simulink model "ProiectSCPC_Reglare_Nivel"  (R2023a)
settings: Solver=FixedStepAuto  StartTime=0.0  StopTime=1000  FixedStep=0.01  RelTol=1e-3
undefined symbols (not defined in the file): C, k, k1, k11, k12, k13, k2, k3, keta
libraries: slpidlib x8
settings Model: Creator=Cristian  LastModifiedBy=Cristian

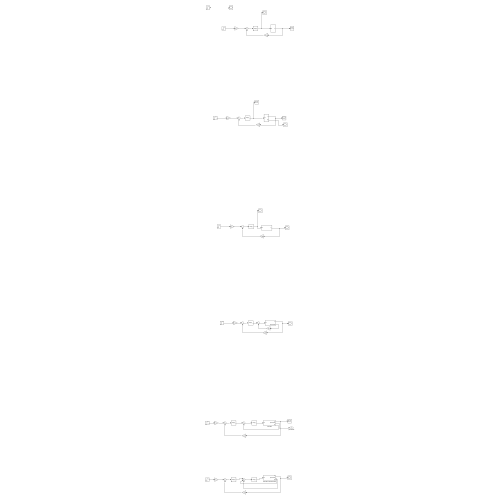
[thumbnail: Simulink's stored preview of the top-level diagram]
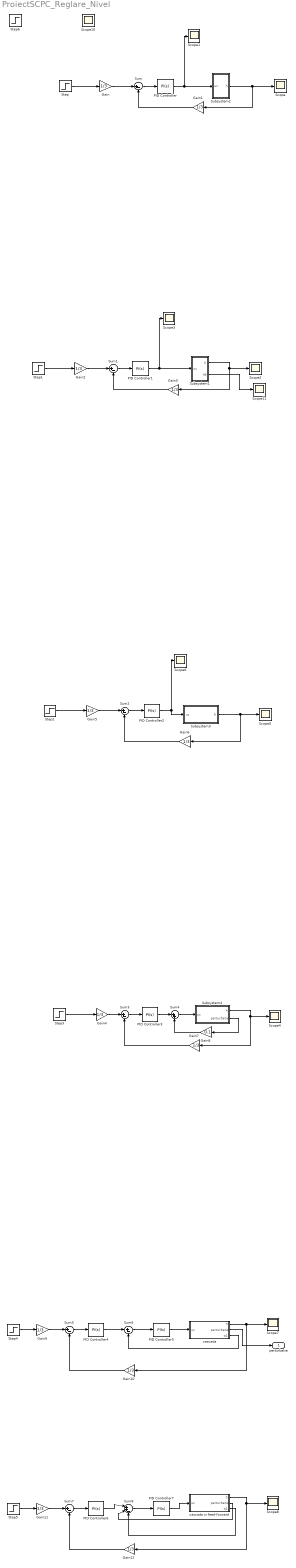
== system ProiectSCPC_Reglare_Nivel ==
  Gain{,1..7,9..12} (12 alike) : Gain  Gain=1/3
  Gain8 : Gain  Gain=0.1
  PID Controller{,1..3} (4 alike) : slpidlib/PID Controller  Controller=PI  Form=Parallel  TimeDomain=Continuous-time  UseExternalTs=off  SampleTime=-1  IntegratorMethod=Forward Euler  FilterMethod=Forward Euler  ControllerParametersSource=internal  P=2.395  I=2.395/160  UseKiTs=off  D=0  N=100  UseFilter=on  TunerSelectOption=Transfer Function Based (PID Tuner App)  InitialConditionSource=internal  InitialConditionForIntegrator=5  InitialConditionForFilter=0  DifferentiatorICPrevScaledInput=0  ExternalReset=none  TrackingMode=off  Kt=1  LimitOutput=off  SatLimitsSource=internal  UpperSaturationLimit=inf  LowerSaturationLimit=-inf  LinearizeAsGain=on  AntiWindupMode=none  Kb=1  LimitIntegrator=off  UpperIntegratorSaturationLimit=inf  LowerIntegratorSaturationLimit=-inf  POutMin=[]  POutMax=[]  IOutMin=[]  IOutMax=[]  DOutMin=[]  DOutMax=[]  NOutMin=[]  NOutMax=[]  SumOutMin=[]  SumOutMax=[]  SaturationOutMin=[]  SaturationOutMax=[]  PParamMin=[]  PParamMax=[]  IParamMin=[]  IParamMax=[]  DParamMin=[]  DParamMax=[]  NParamMin=[]  NParamMax=[]  KbParamMin=[]  KbParamMax=[]  KtParamMin=[]  KtParamMax=[]  KbOutMin=[]  KbOutMax=[]  KtOutMin=[]  KtOutMax=[]  IntegratorOutMin=[]  IntegratorOutMax=[]  FilterOutMin=[]  FilterOutMax=[]  SumI1OutMin=[]  SumI1OutMax=[]  SumI2OutMin=[]  SumI2OutMax=[]  SumI3OutMin=[]  SumI3OutMax=[]  SumI4OutMin=[]  SumI4OutMax=[]  SumDOutMin=[]  SumDOutMax=[]  DifferentiatorOutMin=[]  DifferentiatorOutMax=[]  FilterDiffOutCoefMin=[]  FilterDiffOutCoefMax=[]  ReciprocalOutMin=[]  ReciprocalOutMax=[]  SumDenOutMin=[]  SumDenOutMax=[]  SumNumOutMin=[]  SumNumOutMax=[]  DivideOutMin=[]  DivideOutMax=[]  UdiffTsProdOutMin=[]  UdiffTsProdOutMax=[]  NTsProdOutMin=[]  NTsProdOutMax=[]  UintegralTsProdOutMin=[]  UintegralTsProdOutMax=[]  UngainTsProdOutMin=[]  UngainTsProdOutMax=[]  ClampingZeroOutDataTypeStr=Inherit: Inherit via back propagation  ClampingZeroOutMin=[]  ClampingZeroOutMax=[]  FilterDenConstantOutDataTypeStr=Inherit: Inherit via back propagation  FilterDenConstantOutMin=[]  FilterDenConstantOutMax=[]  PCopyOutDataTypeStr=Inherit: Inherit via back propagation  PCopyOutMin=[]  PCopyOutMax=[]  NCopyOutDataTypeStr=Inherit: Inherit via back propagation  NCopyOutMin=[]  NCopyOutMax=[]  IntegratorContinuousStateAttributes=''  IntegratorStateMustResolveToSignalObject=off  IntegratorRTWStateStorageClass=Auto  FilterContinuousStateAttributes=''  FilterStateMustResolveToSignalObject=off  FilterRTWStateStorageClass=Auto  ParallelPVariant=InternalParameters  IdealPVariant=Disabled  IVariant=InternalParameters  DVariant=Disabled  IntegratorVariant=Continuous  SatVariant=Disabled  AWVariant=Passthrough  PCopyVariant=Disabled  TRVariant=Disabled  FdbkBlocksVariant=Forward  IdealPFdbkVariant=Disabled  SatFdbkVariant=Disabled  DerivativeFilterVariant=Disabled  NVariant=Disabled  NCopyVariant=Disabled_SignalSpec  FilterICVariant=Disabled  IntegratorICVariant=InternalICs  ExternalResetVariant=Disabled  TRSumVariant=Passthrough  SumFdbkVariant=Disabled  SumVariant=Sum_PI  TsampFilterVariant=InternalTs  TsampNgainVariant=Passthrough  TsampIntegralVariant=Disabled_SignalSpec  ExternalSaturationOutDataTypeStr=Inherit: Same as second input
  PID Controller4 : slpidlib/PID Controller  Controller=PI  Form=Parallel  TimeDomain=Continuous-time  UseExternalTs=off  SampleTime=-1  IntegratorMethod=Forward Euler  FilterMethod=Forward Euler  ControllerParametersSource=internal  P=39  I=0.16  UseKiTs=off  D=0  N=100  UseFilter=on  TunerSelectOption=Transfer Function Based (PID Tuner App)  InitialConditionSource=internal  InitialConditionForIntegrator=29.2  InitialConditionForFilter=0  DifferentiatorICPrevScaledInput=0  ExternalReset=none  TrackingMode=off  Kt=1  LimitOutput=off  SatLimitsSource=internal  UpperSaturationLimit=inf  LowerSaturationLimit=-inf  LinearizeAsGain=on  AntiWindupMode=none  Kb=1  LimitIntegrator=off  UpperIntegratorSaturationLimit=inf  LowerIntegratorSaturationLimit=-inf  POutMin=[]  POutMax=[]  IOutMin=[]  IOutMax=[]  DOutMin=[]  DOutMax=[]  NOutMin=[]  NOutMax=[]  SumOutMin=[]  SumOutMax=[]  SaturationOutMin=[]  SaturationOutMax=[]  PParamMin=[]  PParamMax=[]  IParamMin=[]  IParamMax=[]  DParamMin=[]  DParamMax=[]  NParamMin=[]  NParamMax=[]  KbParamMin=[]  KbParamMax=[]  KtParamMin=[]  KtParamMax=[]  KbOutMin=[]  KbOutMax=[]  KtOutMin=[]  KtOutMax=[]  IntegratorOutMin=[]  IntegratorOutMax=[]  FilterOutMin=[]  FilterOutMax=[]  SumI1OutMin=[]  SumI1OutMax=[]  SumI2OutMin=[]  SumI2OutMax=[]  SumI3OutMin=[]  SumI3OutMax=[]  SumI4OutMin=[]  SumI4OutMax=[]  SumDOutMin=[]  SumDOutMax=[]  DifferentiatorOutMin=[]  DifferentiatorOutMax=[]  FilterDiffOutCoefMin=[]  FilterDiffOutCoefMax=[]  ReciprocalOutMin=[]  ReciprocalOutMax=[]  SumDenOutMin=[]  SumDenOutMax=[]  SumNumOutMin=[]  SumNumOutMax=[]  DivideOutMin=[]  DivideOutMax=[]  UdiffTsProdOutMin=[]  UdiffTsProdOutMax=[]  NTsProdOutMin=[]  NTsProdOutMax=[]  UintegralTsProdOutMin=[]  UintegralTsProdOutMax=[]  UngainTsProdOutMin=[]  UngainTsProdOutMax=[]  ClampingZeroOutDataTypeStr=Inherit: Inherit via back propagation  ClampingZeroOutMin=[]  ClampingZeroOutMax=[]  FilterDenConstantOutDataTypeStr=Inherit: Inherit via back propagation  FilterDenConstantOutMin=[]  FilterDenConstantOutMax=[]  PCopyOutDataTypeStr=Inherit: Inherit via back propagation  PCopyOutMin=[]  PCopyOutMax=[]  NCopyOutDataTypeStr=Inherit: Inherit via back propagation  NCopyOutMin=[]  NCopyOutMax=[]  IntegratorContinuousStateAttributes=''  IntegratorStateMustResolveToSignalObject=off  IntegratorRTWStateStorageClass=Auto  FilterContinuousStateAttributes=''  FilterStateMustResolveToSignalObject=off  FilterRTWStateStorageClass=Auto  ParallelPVariant=InternalParameters  IdealPVariant=Disabled  IVariant=InternalParameters  DVariant=Disabled  IntegratorVariant=Continuous  SatVariant=Disabled  AWVariant=Passthrough  PCopyVariant=Disabled  TRVariant=Disabled  FdbkBlocksVariant=Forward  IdealPFdbkVariant=Disabled  SatFdbkVariant=Disabled  DerivativeFilterVariant=Disabled  NVariant=Disabled  NCopyVariant=Disabled_SignalSpec  FilterICVariant=Disabled  IntegratorICVariant=InternalICs  ExternalResetVariant=Disabled  TRSumVariant=Passthrough  SumFdbkVariant=Disabled  SumVariant=Sum_PI  TsampFilterVariant=InternalTs  TsampNgainVariant=Passthrough  TsampIntegralVariant=Disabled_SignalSpec  ExternalSaturationOutDataTypeStr=Inherit: Same as second input
  PID Controller5 : slpidlib/PID Controller  Controller=PI  Form=Parallel  TimeDomain=Continuous-time  UseExternalTs=off  SampleTime=-1  IntegratorMethod=Forward Euler  FilterMethod=Forward Euler  ControllerParametersSource=internal  P=0.07  I=1  UseKiTs=off  D=0  N=100  UseFilter=on  TunerSelectOption=Transfer Function Based (PID Tuner App)  InitialConditionSource=internal  InitialConditionForIntegrator=5  InitialConditionForFilter=0  DifferentiatorICPrevScaledInput=0  ExternalReset=none  TrackingMode=off  Kt=1  LimitOutput=off  SatLimitsSource=internal  UpperSaturationLimit=inf  LowerSaturationLimit=-inf  LinearizeAsGain=on  AntiWindupMode=none  Kb=1  LimitIntegrator=off  UpperIntegratorSaturationLimit=inf  LowerIntegratorSaturationLimit=-inf  POutMin=[]  POutMax=[]  IOutMin=[]  IOutMax=[]  DOutMin=[]  DOutMax=[]  NOutMin=[]  NOutMax=[]  SumOutMin=[]  SumOutMax=[]  SaturationOutMin=[]  SaturationOutMax=[]  PParamMin=[]  PParamMax=[]  IParamMin=[]  IParamMax=[]  DParamMin=[]  DParamMax=[]  NParamMin=[]  NParamMax=[]  KbParamMin=[]  KbParamMax=[]  KtParamMin=[]  KtParamMax=[]  KbOutMin=[]  KbOutMax=[]  KtOutMin=[]  KtOutMax=[]  IntegratorOutMin=[]  IntegratorOutMax=[]  FilterOutMin=[]  FilterOutMax=[]  SumI1OutMin=[]  SumI1OutMax=[]  SumI2OutMin=[]  SumI2OutMax=[]  SumI3OutMin=[]  SumI3OutMax=[]  SumI4OutMin=[]  SumI4OutMax=[]  SumDOutMin=[]  SumDOutMax=[]  DifferentiatorOutMin=[]  DifferentiatorOutMax=[]  FilterDiffOutCoefMin=[]  FilterDiffOutCoefMax=[]  ReciprocalOutMin=[]  ReciprocalOutMax=[]  SumDenOutMin=[]  SumDenOutMax=[]  SumNumOutMin=[]  SumNumOutMax=[]  DivideOutMin=[]  DivideOutMax=[]  UdiffTsProdOutMin=[]  UdiffTsProdOutMax=[]  NTsProdOutMin=[]  NTsProdOutMax=[]  UintegralTsProdOutMin=[]  UintegralTsProdOutMax=[]  UngainTsProdOutMin=[]  UngainTsProdOutMax=[]  ClampingZeroOutDataTypeStr=Inherit: Inherit via back propagation  ClampingZeroOutMin=[]  ClampingZeroOutMax=[]  FilterDenConstantOutDataTypeStr=Inherit: Inherit via back propagation  FilterDenConstantOutMin=[]  FilterDenConstantOutMax=[]  PCopyOutDataTypeStr=Inherit: Inherit via back propagation  PCopyOutMin=[]  PCopyOutMax=[]  NCopyOutDataTypeStr=Inherit: Inherit via back propagation  NCopyOutMin=[]  NCopyOutMax=[]  IntegratorContinuousStateAttributes=''  IntegratorStateMustResolveToSignalObject=off  IntegratorRTWStateStorageClass=Auto  FilterContinuousStateAttributes=''  FilterStateMustResolveToSignalObject=off  FilterRTWStateStorageClass=Auto  ParallelPVariant=InternalParameters  IdealPVariant=Disabled  IVariant=InternalParameters  DVariant=Disabled  IntegratorVariant=Continuous  SatVariant=Disabled  AWVariant=Passthrough  PCopyVariant=Disabled  TRVariant=Disabled  FdbkBlocksVariant=Forward  IdealPFdbkVariant=Disabled  SatFdbkVariant=Disabled  DerivativeFilterVariant=Disabled  NVariant=Disabled  NCopyVariant=Disabled_SignalSpec  FilterICVariant=Disabled  IntegratorICVariant=InternalICs  ExternalResetVariant=Disabled  TRSumVariant=Passthrough  SumFdbkVariant=Disabled  SumVariant=Sum_PI  TsampFilterVariant=InternalTs  TsampNgainVariant=Passthrough  TsampIntegralVariant=Disabled_SignalSpec  ExternalSaturationOutDataTypeStr=Inherit: Same as second input
  PID Controller6 : slpidlib/PID Controller  Controller=PI  Form=Parallel  TimeDomain=Continuous-time  UseExternalTs=off  SampleTime=-1  IntegratorMethod=Forward Euler  FilterMethod=Forward Euler  ControllerParametersSource=internal  P=40  I=40/250  UseKiTs=off  D=0  N=100  UseFilter=on  TunerSelectOption=Transfer Function Based (PID Tuner App)  InitialConditionSource=internal  InitialConditionForIntegrator=29.2  InitialConditionForFilter=0  DifferentiatorICPrevScaledInput=0  ExternalReset=none  TrackingMode=off  Kt=1  LimitOutput=off  SatLimitsSource=internal  UpperSaturationLimit=inf  LowerSaturationLimit=-inf  LinearizeAsGain=on  AntiWindupMode=none  Kb=1  LimitIntegrator=off  UpperIntegratorSaturationLimit=inf  LowerIntegratorSaturationLimit=-inf  POutMin=[]  POutMax=[]  IOutMin=[]  IOutMax=[]  DOutMin=[]  DOutMax=[]  NOutMin=[]  NOutMax=[]  SumOutMin=[]  SumOutMax=[]  SaturationOutMin=[]  SaturationOutMax=[]  PParamMin=[]  PParamMax=[]  IParamMin=[]  IParamMax=[]  DParamMin=[]  DParamMax=[]  NParamMin=[]  NParamMax=[]  KbParamMin=[]  KbParamMax=[]  KtParamMin=[]  KtParamMax=[]  KbOutMin=[]  KbOutMax=[]  KtOutMin=[]  KtOutMax=[]  IntegratorOutMin=[]  IntegratorOutMax=[]  FilterOutMin=[]  FilterOutMax=[]  SumI1OutMin=[]  SumI1OutMax=[]  SumI2OutMin=[]  SumI2OutMax=[]  SumI3OutMin=[]  SumI3OutMax=[]  SumI4OutMin=[]  SumI4OutMax=[]  SumDOutMin=[]  SumDOutMax=[]  DifferentiatorOutMin=[]  DifferentiatorOutMax=[]  FilterDiffOutCoefMin=[]  FilterDiffOutCoefMax=[]  ReciprocalOutMin=[]  ReciprocalOutMax=[]  SumDenOutMin=[]  SumDenOutMax=[]  SumNumOutMin=[]  SumNumOutMax=[]  DivideOutMin=[]  DivideOutMax=[]  UdiffTsProdOutMin=[]  UdiffTsProdOutMax=[]  NTsProdOutMin=[]  NTsProdOutMax=[]  UintegralTsProdOutMin=[]  UintegralTsProdOutMax=[]  UngainTsProdOutMin=[]  UngainTsProdOutMax=[]  ClampingZeroOutDataTypeStr=Inherit: Inherit via back propagation  ClampingZeroOutMin=[]  ClampingZeroOutMax=[]  FilterDenConstantOutDataTypeStr=Inherit: Inherit via back propagation  FilterDenConstantOutMin=[]  FilterDenConstantOutMax=[]  PCopyOutDataTypeStr=Inherit: Inherit via back propagation  PCopyOutMin=[]  PCopyOutMax=[]  NCopyOutDataTypeStr=Inherit: Inherit via back propagation  NCopyOutMin=[]  NCopyOutMax=[]  IntegratorContinuousStateAttributes=''  IntegratorStateMustResolveToSignalObject=off  IntegratorRTWStateStorageClass=Auto  FilterContinuousStateAttributes=''  FilterStateMustResolveToSignalObject=off  FilterRTWStateStorageClass=Auto  ParallelPVariant=InternalParameters  IdealPVariant=Disabled  IVariant=InternalParameters  DVariant=Disabled  IntegratorVariant=Continuous  SatVariant=Disabled  AWVariant=Passthrough  PCopyVariant=Disabled  TRVariant=Disabled  FdbkBlocksVariant=Forward  IdealPFdbkVariant=Disabled  SatFdbkVariant=Disabled  DerivativeFilterVariant=Disabled  NVariant=Disabled  NCopyVariant=Disabled_SignalSpec  FilterICVariant=Disabled  IntegratorICVariant=InternalICs  ExternalResetVariant=Disabled  TRSumVariant=Passthrough  SumFdbkVariant=Disabled  SumVariant=Sum_PI  TsampFilterVariant=InternalTs  TsampNgainVariant=Passthrough  TsampIntegralVariant=Disabled_SignalSpec  ExternalSaturationOutDataTypeStr=Inherit: Same as second input
  PID Controller7 : slpidlib/PID Controller  Controller=PI  Form=Parallel  TimeDomain=Continuous-time  UseExternalTs=off  SampleTime=-1  IntegratorMethod=Forward Euler  FilterMethod=Forward Euler  ControllerParametersSource=internal  P=0.07  I=1  UseKiTs=off  D=0  N=100  UseFilter=on  TunerSelectOption=Transfer Function Based (PID Tuner App)  InitialConditionSource=internal  InitialConditionForIntegrator=5  InitialConditionForFilter=0  DifferentiatorICPrevScaledInput=0  ExternalReset=none  TrackingMode=off  Kt=1  LimitOutput=off  SatLimitsSource=internal  UpperSaturationLimit=inf  LowerSaturationLimit=-inf  LinearizeAsGain=on  AntiWindupMode=none  Kb=1  LimitIntegrator=off  UpperIntegratorSaturationLimit=inf  LowerIntegratorSaturationLimit=-inf  POutMin=[]  POutMax=[]  IOutMin=[]  IOutMax=[]  DOutMin=[]  DOutMax=[]  NOutMin=[]  NOutMax=[]  SumOutMin=[]  SumOutMax=[]  SaturationOutMin=[]  SaturationOutMax=[]  PParamMin=[]  PParamMax=[]  IParamMin=[]  IParamMax=[]  DParamMin=[]  DParamMax=[]  NParamMin=[]  NParamMax=[]  KbParamMin=[]  KbParamMax=[]  KtParamMin=[]  KtParamMax=[]  KbOutMin=[]  KbOutMax=[]  KtOutMin=[]  KtOutMax=[]  IntegratorOutMin=[]  IntegratorOutMax=[]  FilterOutMin=[]  FilterOutMax=[]  SumI1OutMin=[]  SumI1OutMax=[]  SumI2OutMin=[]  SumI2OutMax=[]  SumI3OutMin=[]  SumI3OutMax=[]  SumI4OutMin=[]  SumI4OutMax=[]  SumDOutMin=[]  SumDOutMax=[]  DifferentiatorOutMin=[]  DifferentiatorOutMax=[]  FilterDiffOutCoefMin=[]  FilterDiffOutCoefMax=[]  ReciprocalOutMin=[]  ReciprocalOutMax=[]  SumDenOutMin=[]  SumDenOutMax=[]  SumNumOutMin=[]  SumNumOutMax=[]  DivideOutMin=[]  DivideOutMax=[]  UdiffTsProdOutMin=[]  UdiffTsProdOutMax=[]  NTsProdOutMin=[]  NTsProdOutMax=[]  UintegralTsProdOutMin=[]  UintegralTsProdOutMax=[]  UngainTsProdOutMin=[]  UngainTsProdOutMax=[]  ClampingZeroOutDataTypeStr=Inherit: Inherit via back propagation  ClampingZeroOutMin=[]  ClampingZeroOutMax=[]  FilterDenConstantOutDataTypeStr=Inherit: Inherit via back propagation  FilterDenConstantOutMin=[]  FilterDenConstantOutMax=[]  PCopyOutDataTypeStr=Inherit: Inherit via back propagation  PCopyOutMin=[]  PCopyOutMax=[]  NCopyOutDataTypeStr=Inherit: Inherit via back propagation  NCopyOutMin=[]  NCopyOutMax=[]  IntegratorContinuousStateAttributes=''  IntegratorStateMustResolveToSignalObject=off  IntegratorRTWStateStorageClass=Auto  FilterContinuousStateAttributes=''  FilterStateMustResolveToSignalObject=off  FilterRTWStateStorageClass=Auto  ParallelPVariant=InternalParameters  IdealPVariant=Disabled  IVariant=InternalParameters  DVariant=Disabled  IntegratorVariant=Continuous  SatVariant=Disabled  AWVariant=Passthrough  PCopyVariant=Disabled  TRVariant=Disabled  FdbkBlocksVariant=Forward  IdealPFdbkVariant=Disabled  SatFdbkVariant=Disabled  DerivativeFilterVariant=Disabled  NVariant=Disabled  NCopyVariant=Disabled_SignalSpec  FilterICVariant=Disabled  IntegratorICVariant=InternalICs  ExternalResetVariant=Disabled  TRSumVariant=Passthrough  SumFdbkVariant=Disabled  SumVariant=Sum_PI  TsampFilterVariant=InternalTs  TsampNgainVariant=Passthrough  TsampIntegralVariant=Disabled_SignalSpec  ExternalSaturationOutDataTypeStr=Inherit: Same as second input
  Scope{,1..8,10..11} (11 alike) : Scope
  Step{,1..3} (4 alike) : Step  Time=0  Before=10.5  After=13  SampleTime=0
  Step4 : Step  Before=10.51  After=13  SampleTime=0
  Step5 : Step  Before=10.51  After=13  SampleTime=0
  Step6 : Step  Time=0  Before=5  After=5.5  SampleTime=0
  Subsystem1 : Subsystem
  Subsystem2 : Subsystem
  Subsystem3 : Subsystem
  Subsystem4 : Subsystem
  Sum{,1..3,5..7} (7 alike) : Sum  Inputs=|+-
  Sum4 : Sum  Inputs=|++
  Sum8 : Sum  Inputs=|++-
  cascada : Subsystem
  cascada si feed-forward : Subsystem
  perturbatie : Outport
  wires:
  Subsystem2/1(h) -> Gain1/1, Scope/1
  Gain/1 -> Sum/1
  Sum/1 -> PID Controller/1
  Gain1/1 -> Sum/2
  PID Controller/1 -> Subsystem2/1(uc), Scope1/1
  Step/1 -> Gain/1
  Sum1/1 -> PID Controller1/1
  Step1/1 -> Gain2/1
  Subsystem1/2(qe) -> Scope11/1
  Subsystem1/1(h) -> Gain3/1, Scope2/1
  Gain3/1 -> Sum1/2
  PID Controller1/1 -> Subsystem1/1(uc), Scope3/1
  Gain2/1 -> Sum1/1
  PID Controller2/1 -> Scope6/1, Subsystem3/1(uc)
  Gain6/1 -> Sum2/2
  Sum2/1 -> PID Controller2/1
  Sum3/1 -> PID Controller3/1
  Subsystem4/1(h) -> Gain7/1, Scope4/1
  Step2/1 -> Gain5/1
  Gain7/1 -> Sum3/2
  Step3/1 -> Gain4/1
  PID Controller3/1 -> Sum4/1
  Subsystem4/2(perturbatie) -> Gain8/1
  Gain5/1 -> Sum2/1
  Gain8/1 -> Sum4/2
  Sum4/1 -> Subsystem4/1(uc)
  Subsystem3/1(h) -> Scope5/1, Gain6/1
  Gain4/1 -> Sum3/1
  cascada/1("h ") -> Scope7/1, Gain10/1
  PID Controller4/1 -> Sum6/1
  PID Controller5/1 -> cascada/1(uc)
  Gain10/1 -> Sum5/2
  Gain9/1 -> Sum5/1
  Step4/1 -> Gain9/1
  cascada/3(q1) -> Sum6/2
  Sum6/1 -> PID Controller5/1
  Sum5/1 -> PID Controller4/1
  cascada/2(perturbatie) -> perturbatie/1
  Gain12/1 -> Sum7/2
  cascada si feed-forward/2(perturbatie) -> Sum8/2
  Gain11/1 -> Sum7/1
  Sum7/1 -> PID Controller6/1
  Sum8/1 -> PID Controller7/1
  Step5/1 -> Gain11/1
  cascada si feed-forward/3(q1) -> Sum8/3
  cascada si feed-forward/1("h ") -> Scope8/1, Gain12/1
  PID Controller7/1 -> cascada si feed-forward/1(uc)
  PID Controller6/1 -> Sum8/1

== system ProiectSCPC_Reglare_Nivel/Subsystem1 ==
  uc : Inport
  Amplificator : Subsystem
  Bazin : Subsystem
  Curent : Subsystem
  Motor : Subsystem
  Pompa : Subsystem
  Randament : Subsystem
  Subsystem : Subsystem
  h : Outport
  qe : Outport  Port=2
  wires:
  Randament/1(eta) -> Curent/3(eta)
  Subsystem/1(h) -> Bazin/1(q), Randament/1(q), Curent/2(q)
  Amplificator/1(um) -> Curent/4(um), Randament/2(um), Motor/1(um)
  uc/1 -> Amplificator/1(ua)
  Curent/1(im) -> Motor/2(im)
  Bazin/1(h) -> h/1, Curent/1(h), Pompa/2(h)
  Motor/1(kn) -> Pompa/1(kn)
  Pompa/1(q) -> Subsystem/1(q)
  Bazin/2(qe) -> qe/1

== system ProiectSCPC_Reglare_Nivel/Subsystem2 ==
  uc : Inport
  Amplificator : Subsystem
  Bazin : Subsystem
  Curent : Subsystem
  Motor : Subsystem
  Pompa : Subsystem
  Randament : Subsystem
  Subsystem : Subsystem
  h : Outport
  wires:
  Randament/1(eta) -> Curent/3(eta)
  Subsystem/1(h) -> Bazin/1(q), Randament/1(q), Curent/2(q)
  Amplificator/1(um) -> Curent/4(um), Randament/2(um), Motor/1(um)
  uc/1 -> Amplificator/1(ua)
  Curent/1(im) -> Motor/2(im)
  Bazin/1(h) -> h/1, Curent/1(h), Pompa/2(h)
  Motor/1(kn) -> Pompa/1(kn)
  Pompa/1(q) -> Subsystem/1(q)

== system ProiectSCPC_Reglare_Nivel/Subsystem3 ==
  uc : Inport
  Amplificator : Subsystem
  Bazin : Subsystem
  Curent : Subsystem
  Motor : Subsystem
  Pompa : Subsystem
  Randament : Subsystem
  Step : Step  Time=250  After=0.01  SampleTime=0
  Subsystem : Subsystem
  h : Outport
  wires:
  Motor/1(kn) -> Pompa/1(kn1)
  Subsystem/1(h) -> Bazin/1(q), Randament/1(q), Curent/2(q)
  Pompa/1(q1) -> Subsystem/1(q)
  Randament/1(eta) -> Curent/3(eta)
  Curent/1(im) -> Motor/2(im)
  Bazin/1(h) -> h/1, Pompa/3(h1), Curent/1(h)
  uc/1 -> Amplificator/1(ua)
  Amplificator/1(um) -> Curent/4(um), Randament/2(um), Motor/1(um)
  Step/1 -> Pompa/2(perturbatie k)

== system ProiectSCPC_Reglare_Nivel/Subsystem4 ==
  uc : Inport
  Amplificator : Subsystem
  Bazin : Subsystem
  Curent : Subsystem
  Motor : Subsystem
  Pompa : Subsystem
  Randament : Subsystem
  Subsystem : Subsystem
  h : Outport
  perturbatie : Outport  Port=2
  wires:
  Motor/1(kn) -> Pompa/1(kn1)
  Subsystem/1(h) -> Bazin/1(q), Randament/1(q), Curent/2(q)
  Pompa/1(q1) -> Subsystem/1(q)
  Randament/1(eta) -> Curent/3(eta)
  Curent/1(im) -> Motor/2(im)
  Bazin/1(h) -> h/1, Pompa/3(h1), Curent/1(h)
  uc/1 -> Amplificator/1(ua)
  Amplificator/1(um) -> Curent/4(um), Randament/2(um), Motor/1(um)
  Bazin/3(perturbatie) -> perturbatie/1

== system ProiectSCPC_Reglare_Nivel/cascada ==
  uc : Inport
  "Amplificator " : Subsystem
  Curent rotoric : Subsystem
  Filtru : Subsystem
  Motor : Subsystem
  Pompa : Subsystem
  Randament : Subsystem
  Rezervor : Subsystem
  Step : Step  Time=300  After=0.02  SampleTime=0
  "h " : Outport
  perturbatie : Outport  Port=2
  q1 : Outport  Port=3
  wires:
  Filtru/1(h) -> Curent rotoric/1(q), q1/1, Randament/1(q), Rezervor/1(q)
  uc/1 -> "Amplificator "/1(ua)
  Randament/1(eta) -> Curent rotoric/2(eta)
  Rezervor/1(h) -> Curent rotoric/3(h), Pompa/2(h1), "h "/1
  Pompa/1(q1) -> Filtru/1(q)
  Curent rotoric/1(im) -> Motor/2(im)
  "Amplificator "/1(um) -> Curent rotoric/4(um), Randament/2(um), Motor/1(um)
  Motor/1(kn) -> Pompa/1(kn1)
  Step/1 -> perturbatie/1, Pompa/3(perturbatie k)

== system ProiectSCPC_Reglare_Nivel/cascada si feed-forward ==
  uc : Inport
  "Amplificator " : Subsystem
  Curent rotoric : Subsystem
  Filtru : Subsystem
  Motor : Subsystem
  Pompa : Subsystem
  Randament : Subsystem
  Rezervor : Subsystem
  Step : Step  Time=300  After=-.035  SampleTime=0
  "h " : Outport
  perturbatie : Outport  Port=2
  q1 : Outport  Port=3
  wires:
  Filtru/1(h) -> Curent rotoric/1(q), q1/1, Randament/1(q), Rezervor/1(q)
  uc/1 -> "Amplificator "/1(ua)
  Randament/1(eta) -> Curent rotoric/2(eta)
  Rezervor/1(h) -> Curent rotoric/3(h), Pompa/2(h1), "h "/1
  Pompa/1(q1) -> Filtru/1(q)
  Curent rotoric/1(im) -> Motor/2(im)
  "Amplificator "/1(um) -> Curent rotoric/4(um), Randament/2(um), Motor/1(um)
  Motor/1(kn) -> Pompa/1(kn1)
  Step/1 -> perturbatie/1, Pompa/3(perturbatie k)

== system ProiectSCPC_Reglare_Nivel/Subsystem1/Amplificator ==
  ua : Inport
  Constant : Constant  Value=8.1
  Gain : Gain  Gain=2.2
  Gain1 : Gain  Gain=5
  Gain2 : Gain  Gain=2.2
  Saturation : Saturate  UpperLimit=22  LowerLimit=0
  Sum : Sum  Inputs=|+-
  Sum1 : Sum  Inputs=|++
  Switch : Switch  Threshold=8.1  SaturateOnIntegerOverflow=off  InputSameDT=off
  um : Outport
  wires:
  ua/1 -> Gain/1, Switch/2, Sum/1, Gain2/1
  Gain1/1 -> Sum1/2
  Saturation/1 -> um/1
  Switch/1 -> Saturation/1
  Constant/1 -> Sum/2
  Gain/1 -> Switch/3
  Sum1/1 -> Switch/1
  Sum/1 -> Gain1/1
  Gain2/1 -> Sum1/1

== system ProiectSCPC_Reglare_Nivel/Subsystem1/Bazin ==
  q : Inport
  Gain12 : Gain  Gain=1/332.5
  Integrator : Integrator  InitialCondition=10.5
  Product : Product
  Sqrt : Sqrt
  Step : Step  Time=250  Before=9  After=11  SampleTime=0
  Sum2 : Sum  Inputs=|+-
  h : Outport
  qe : Outport  Port=2
  wires:
  Sum2/1 -> Gain12/1
  Gain12/1 -> Integrator/1
  q/1 -> Sum2/1
  Integrator/1 -> Sqrt/1, h/1
  Product/1 -> qe/1, Sum2/2
  Sqrt/1 -> Product/1
  Step/1 -> Product/2

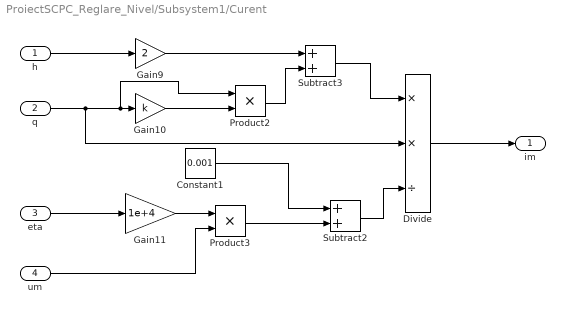
== system ProiectSCPC_Reglare_Nivel/Subsystem1/Curent ==
  h : Inport
  q : Inport  Port=2
  eta : Inport  Port=3
  um : Inport  Port=4
  Constant1 : Constant  Value=0.001
  Divide : Product  Inputs=**/
  Gain10 : Gain  Gain=k
  Gain11 : Gain  Gain=1e+4
  Gain9 : Gain  Gain=2
  Product2 : Product
  Product3 : Product
  Subtract2 : Sum
  Subtract3 : Sum
  im : Outport
  wires:
  h/1 -> Gain9/1
  q/1 -> Divide/2, Product2/1, Gain10/1
  Gain9/1 -> Subtract3/1
  Product2/1 -> Subtract3/2
  eta/1 -> Gain11/1
  Gain10/1 -> Product2/2
  Subtract2/1 -> Divide/3
  um/1 -> Product3/2
  Gain11/1 -> Product3/1
  Product3/1 -> Subtract2/2
  Constant1/1 -> Subtract2/1
  Divide/1 -> im/1
  Subtract3/1 -> Divide/1

== system ProiectSCPC_Reglare_Nivel/Subsystem1/Motor ==
  um : Inport
  im : Inport  Port=2
  Add : Sum  Inputs=+-
  Gain3 : Gain  Gain=3
  kn : Outport
  wires:
  Gain3/1 -> Add/2
  im/1 -> Gain3/1
  um/1 -> Add/1
  Add/1 -> kn/1

== system ProiectSCPC_Reglare_Nivel/Subsystem1/Pompa ==
  kn : Inport
  h : Inport  Port=2
  Gain4 : Gain  Gain=k2
  Gain5 : Gain  Gain=k11
  Gain6 : Gain  Gain=k12
  Gain7 : Gain  Gain=1/k13
  Product : Product
  Sqrt : Sqrt
  Subtract : Sum  Inputs=+-
  Subtract1 : Sum
  q : Outport
  wires:
  Subtract1/1 -> Gain7/1
  kn/1 -> Gain4/1, Product/1, Product/2
  Sqrt/1 -> Subtract1/2
  h/1 -> Gain6/1
  Product/1 -> Gain5/1
  Gain4/1 -> Subtract1/1
  Gain7/1 -> q/1
  Subtract/1 -> Sqrt/1
  Gain6/1 -> Subtract/2
  Gain5/1 -> Subtract/1

== system ProiectSCPC_Reglare_Nivel/Subsystem1/Randament ==
  q : Inport
  um : Inport  Port=2
  Gain8 : Gain  Gain=keta
  Product1 : Product
  eta : Outport
  wires:
  um/1 -> Gain8/1
  Gain8/1 -> Product1/2
  q/1 -> Product1/1
  Product1/1 -> eta/1

== system ProiectSCPC_Reglare_Nivel/Subsystem1/Subsystem ==
  q : Inport
  Integrator : Integrator  InitialCondition=29.2
  Sum : Sum  Inputs=|+-
  h : Outport
  wires:
  q/1 -> Sum/1
  Integrator/1 -> h/1, Sum/2
  Sum/1 -> Integrator/1

== system ProiectSCPC_Reglare_Nivel/Subsystem2/Amplificator ==
  ua : Inport
  Constant : Constant  Value=8.1
  Gain : Gain  Gain=2.2
  Gain1 : Gain  Gain=5
  Gain2 : Gain  Gain=2.2
  Saturation : Saturate  UpperLimit=22  LowerLimit=0
  Sum : Sum  Inputs=|+-
  Sum1 : Sum  Inputs=|++
  Switch : Switch  Threshold=8.1  SaturateOnIntegerOverflow=off  InputSameDT=off
  um : Outport
  wires:
  ua/1 -> Gain/1, Switch/2, Sum/1, Gain2/1
  Gain1/1 -> Sum1/2
  Saturation/1 -> um/1
  Switch/1 -> Saturation/1
  Constant/1 -> Sum/2
  Gain/1 -> Switch/3
  Sum1/1 -> Switch/1
  Sum/1 -> Gain1/1
  Gain2/1 -> Sum1/1

== system ProiectSCPC_Reglare_Nivel/Subsystem2/Bazin ==
  q : Inport
  Fcn : Fcn  Expr=sqrt(u)*9
  Gain12 : Gain  Gain=1/332.5
  Integrator : Integrator  InitialCondition=10.5
  Sum2 : Sum  Inputs=|+-
  h : Outport
  wires:
  Sum2/1 -> Gain12/1
  Gain12/1 -> Integrator/1
  q/1 -> Sum2/1
  Fcn/1 -> Sum2/2
  Integrator/1 -> Fcn/1, h/1

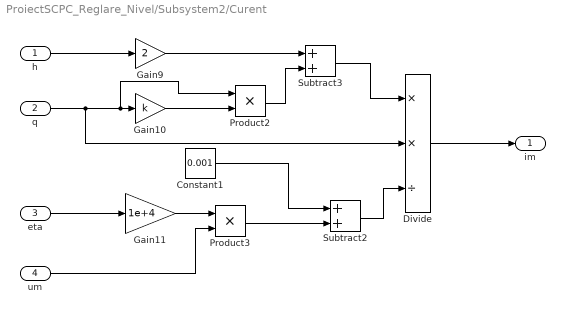
== system ProiectSCPC_Reglare_Nivel/Subsystem2/Curent ==
  h : Inport
  q : Inport  Port=2
  eta : Inport  Port=3
  um : Inport  Port=4
  Constant1 : Constant  Value=0.001
  Divide : Product  Inputs=**/
  Gain10 : Gain  Gain=k
  Gain11 : Gain  Gain=1e+4
  Gain9 : Gain  Gain=2
  Product2 : Product
  Product3 : Product
  Subtract2 : Sum
  Subtract3 : Sum
  im : Outport
  wires:
  h/1 -> Gain9/1
  q/1 -> Divide/2, Product2/1, Gain10/1
  Gain9/1 -> Subtract3/1
  Product2/1 -> Subtract3/2
  eta/1 -> Gain11/1
  Gain10/1 -> Product2/2
  Subtract2/1 -> Divide/3
  um/1 -> Product3/2
  Gain11/1 -> Product3/1
  Product3/1 -> Subtract2/2
  Constant1/1 -> Subtract2/1
  Divide/1 -> im/1
  Subtract3/1 -> Divide/1

== system ProiectSCPC_Reglare_Nivel/Subsystem2/Motor ==
  um : Inport
  im : Inport  Port=2
  Add : Sum  Inputs=+-
  Gain3 : Gain  Gain=3
  kn : Outport
  wires:
  Gain3/1 -> Add/2
  im/1 -> Gain3/1
  um/1 -> Add/1
  Add/1 -> kn/1

== system ProiectSCPC_Reglare_Nivel/Subsystem2/Pompa ==
  kn : Inport
  h : Inport  Port=2
  Gain4 : Gain  Gain=k2
  Gain5 : Gain  Gain=k11
  Gain6 : Gain  Gain=k12
  Gain7 : Gain  Gain=1/k13
  Product : Product
  Sqrt : Sqrt
  Subtract : Sum  Inputs=+-
  Subtract1 : Sum
  q : Outport
  wires:
  Subtract1/1 -> Gain7/1
  kn/1 -> Gain4/1, Product/1, Product/2
  Sqrt/1 -> Subtract1/2
  h/1 -> Gain6/1
  Product/1 -> Gain5/1
  Gain4/1 -> Subtract1/1
  Gain7/1 -> q/1
  Subtract/1 -> Sqrt/1
  Gain6/1 -> Subtract/2
  Gain5/1 -> Subtract/1

== system ProiectSCPC_Reglare_Nivel/Subsystem2/Randament ==
  q : Inport
  um : Inport  Port=2
  Gain8 : Gain  Gain=keta
  Product1 : Product
  eta : Outport
  wires:
  um/1 -> Gain8/1
  Gain8/1 -> Product1/2
  q/1 -> Product1/1
  Product1/1 -> eta/1

== system ProiectSCPC_Reglare_Nivel/Subsystem2/Subsystem ==
  q : Inport
  Integrator : Integrator  InitialCondition=29.2
  Sum : Sum  Inputs=|+-
  h : Outport
  wires:
  q/1 -> Sum/1
  Integrator/1 -> h/1, Sum/2
  Sum/1 -> Integrator/1

== system ProiectSCPC_Reglare_Nivel/Subsystem3/Amplificator ==
  ua : Inport
  Constant : Constant  Value=8.1
  Gain : Gain  Gain=2.2
  Gain1 : Gain  Gain=5
  Gain2 : Gain  Gain=2.2
  Saturation : Saturate  UpperLimit=22  LowerLimit=0
  Sum : Sum  Inputs=|+-
  Sum1 : Sum  Inputs=|++
  Switch : Switch  Threshold=8.1  SaturateOnIntegerOverflow=off  InputSameDT=off
  um : Outport
  wires:
  ua/1 -> Gain/1, Switch/2, Sum/1, Gain2/1
  Gain1/1 -> Sum1/2
  Saturation/1 -> um/1
  Switch/1 -> Saturation/1
  Constant/1 -> Sum/2
  Gain/1 -> Switch/3
  Sum1/1 -> Switch/1
  Sum/1 -> Gain1/1
  Gain2/1 -> Sum1/1

== system ProiectSCPC_Reglare_Nivel/Subsystem3/Bazin ==
  q : Inport
  Gain12 : Gain  Gain=1/332.5
  Integrator : Integrator  InitialCondition=10.5
  Product : Product
  Sqrt : Sqrt
  Step : Step  Time=250  Before=9  After=11  SampleTime=0
  Sum2 : Sum  Inputs=|+-
  h : Outport
  qe : Outport  Port=2
  wires:
  Sum2/1 -> Gain12/1
  Gain12/1 -> Integrator/1
  q/1 -> Sum2/1
  Integrator/1 -> Sqrt/1, h/1
  Product/1 -> qe/1, Sum2/2
  Sqrt/1 -> Product/1
  Step/1 -> Product/2

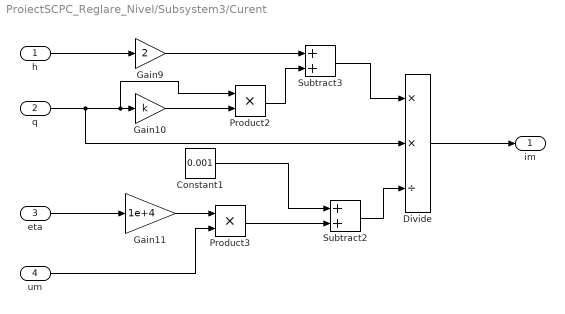
== system ProiectSCPC_Reglare_Nivel/Subsystem3/Curent ==
  h : Inport
  q : Inport  Port=2
  eta : Inport  Port=3
  um : Inport  Port=4
  Constant1 : Constant  Value=0.001
  Divide : Product  Inputs=**/
  Gain10 : Gain  Gain=k
  Gain11 : Gain  Gain=1e+4
  Gain9 : Gain  Gain=2
  Product2 : Product
  Product3 : Product
  Subtract2 : Sum
  Subtract3 : Sum
  im : Outport
  wires:
  h/1 -> Gain9/1
  q/1 -> Divide/2, Product2/1, Gain10/1
  Gain9/1 -> Subtract3/1
  Product2/1 -> Subtract3/2
  eta/1 -> Gain11/1
  Gain10/1 -> Product2/2
  Subtract2/1 -> Divide/3
  um/1 -> Product3/2
  Gain11/1 -> Product3/1
  Product3/1 -> Subtract2/2
  Constant1/1 -> Subtract2/1
  Divide/1 -> im/1
  Subtract3/1 -> Divide/1

== system ProiectSCPC_Reglare_Nivel/Subsystem3/Motor ==
  um : Inport
  im : Inport  Port=2
  Add : Sum  Inputs=+-
  Gain3 : Gain  Gain=3
  kn : Outport
  wires:
  Gain3/1 -> Add/2
  im/1 -> Gain3/1
  um/1 -> Add/1
  Add/1 -> kn/1

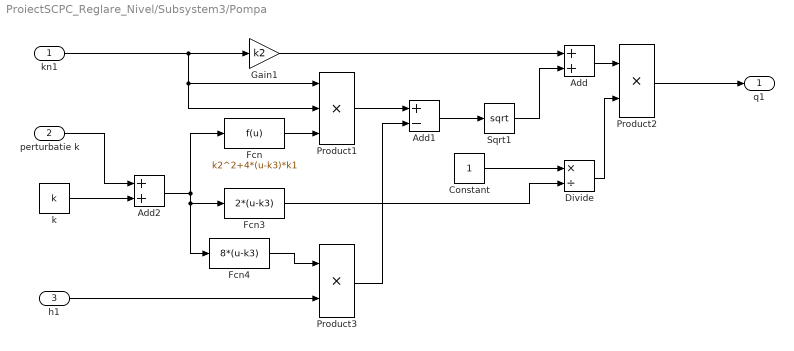
== system ProiectSCPC_Reglare_Nivel/Subsystem3/Pompa ==
  kn1 : Inport
  perturbatie k : Inport  Port=2
  h1 : Inport  Port=3
  Add : Sum
  Add1 : Sum  Inputs=+-
  Add2 : Sum
  Constant : Constant
  Divide : Product  Inputs=*/
  Fcn : Fcn  Expr=k2^2+4*(u-k3)*k1
  Fcn3 : Fcn  Expr=2*(u-k3)
  Fcn4 : Fcn  Expr=8*(u-k3)
  Gain1 : Gain  Gain=k2
  Product1 : Product  Inputs=3
  Product2 : Product
  Product3 : Product
  Sqrt1 : Sqrt
  k : Constant  Value=k
  q1 : Outport
  wires:
  Product3/1 -> Add1/2
  kn1/1 -> Product1/1, Product1/2, Gain1/1
  Constant/1 -> Divide/1
  Fcn3/1 -> Divide/2
  perturbatie k/1 -> Add2/1
  h1/1 -> Product3/2
  k/1 -> Add2/2
  Fcn4/1 -> Product3/1
  Divide/1 -> Product2/2
  Add/1 -> Product2/1
  Product1/1 -> Add1/1
  Product2/1 -> q1/1
  Add1/1 -> Sqrt1/1
  Add2/1 -> Fcn4/1, Fcn3/1, Fcn/1
  Gain1/1 -> Add/1
  Sqrt1/1 -> Add/2
  Fcn/1 -> Product1/3

== system ProiectSCPC_Reglare_Nivel/Subsystem3/Randament ==
  q : Inport
  um : Inport  Port=2
  Gain8 : Gain  Gain=keta
  Product1 : Product
  eta : Outport
  wires:
  um/1 -> Gain8/1
  Gain8/1 -> Product1/2
  q/1 -> Product1/1
  Product1/1 -> eta/1

== system ProiectSCPC_Reglare_Nivel/Subsystem3/Subsystem ==
  q : Inport
  Integrator : Integrator  InitialCondition=29.2
  Sum : Sum  Inputs=|+-
  h : Outport
  wires:
  q/1 -> Sum/1
  Integrator/1 -> h/1, Sum/2
  Sum/1 -> Integrator/1

== system ProiectSCPC_Reglare_Nivel/Subsystem4/Amplificator ==
  ua : Inport
  Constant : Constant  Value=8.1
  Gain : Gain  Gain=2.2
  Gain1 : Gain  Gain=5
  Gain2 : Gain  Gain=2.2
  Saturation : Saturate  UpperLimit=22  LowerLimit=0
  Sum : Sum  Inputs=|+-
  Sum1 : Sum  Inputs=|++
  Switch : Switch  Threshold=8.1  SaturateOnIntegerOverflow=off  InputSameDT=off
  um : Outport
  wires:
  ua/1 -> Gain/1, Switch/2, Sum/1, Gain2/1
  Gain1/1 -> Sum1/2
  Saturation/1 -> um/1
  Switch/1 -> Saturation/1
  Constant/1 -> Sum/2
  Gain/1 -> Switch/3
  Sum1/1 -> Switch/1
  Sum/1 -> Gain1/1
  Gain2/1 -> Sum1/1

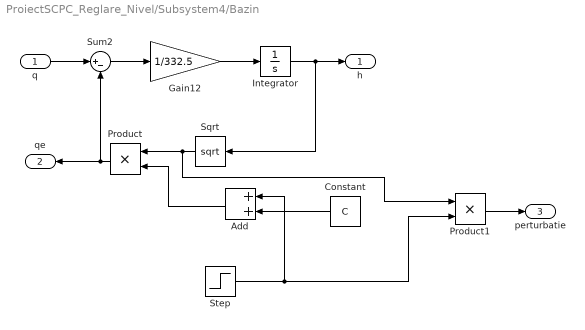
== system ProiectSCPC_Reglare_Nivel/Subsystem4/Bazin ==
  q : Inport
  Add : Sum
  Constant : Constant  Value=C
  Gain12 : Gain  Gain=1/332.5
  Integrator : Integrator  InitialCondition=10.5
  Product : Product
  Product1 : Product
  Sqrt : Sqrt
  Step : Step  Time=500  After=2  SampleTime=0
  Sum2 : Sum  Inputs=|+-
  h : Outport
  qe : Outport  Port=2
  perturbatie : Outport  Port=3
  wires:
  Sum2/1 -> Gain12/1
  Gain12/1 -> Integrator/1
  q/1 -> Sum2/1
  Integrator/1 -> Sqrt/1, h/1
  Product/1 -> qe/1, Sum2/2
  Sqrt/1 -> Product1/1, Product/1
  Add/1 -> Product/2
  Constant/1 -> Add/2
  Step/1 -> Product1/2, Add/1
  Product1/1 -> perturbatie/1

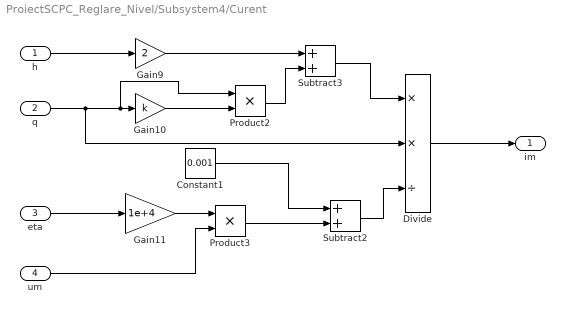
== system ProiectSCPC_Reglare_Nivel/Subsystem4/Curent ==
  h : Inport
  q : Inport  Port=2
  eta : Inport  Port=3
  um : Inport  Port=4
  Constant1 : Constant  Value=0.001
  Divide : Product  Inputs=**/
  Gain10 : Gain  Gain=k
  Gain11 : Gain  Gain=1e+4
  Gain9 : Gain  Gain=2
  Product2 : Product
  Product3 : Product
  Subtract2 : Sum
  Subtract3 : Sum
  im : Outport
  wires:
  h/1 -> Gain9/1
  q/1 -> Divide/2, Product2/1, Gain10/1
  Gain9/1 -> Subtract3/1
  Product2/1 -> Subtract3/2
  eta/1 -> Gain11/1
  Gain10/1 -> Product2/2
  Subtract2/1 -> Divide/3
  um/1 -> Product3/2
  Gain11/1 -> Product3/1
  Product3/1 -> Subtract2/2
  Constant1/1 -> Subtract2/1
  Divide/1 -> im/1
  Subtract3/1 -> Divide/1

== system ProiectSCPC_Reglare_Nivel/Subsystem4/Motor ==
  um : Inport
  im : Inport  Port=2
  Add : Sum  Inputs=+-
  Gain3 : Gain  Gain=3
  kn : Outport
  wires:
  Gain3/1 -> Add/2
  im/1 -> Gain3/1
  um/1 -> Add/1
  Add/1 -> kn/1

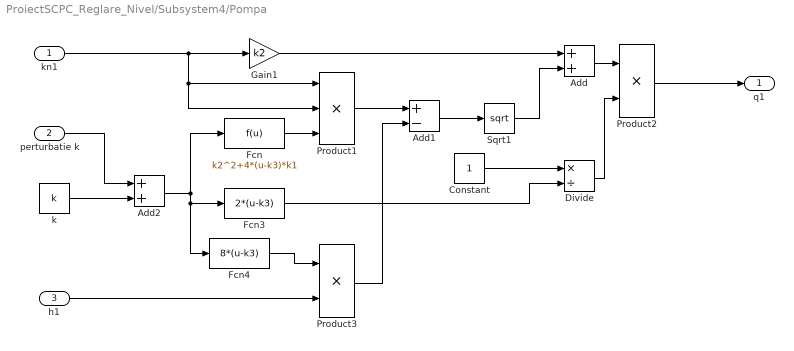
== system ProiectSCPC_Reglare_Nivel/Subsystem4/Pompa ==
  kn1 : Inport
  perturbatie k : Inport  Port=2
  h1 : Inport  Port=3
  Add : Sum
  Add1 : Sum  Inputs=+-
  Add2 : Sum
  Constant : Constant
  Divide : Product  Inputs=*/
  Fcn : Fcn  Expr=k2^2+4*(u-k3)*k1
  Fcn3 : Fcn  Expr=2*(u-k3)
  Fcn4 : Fcn  Expr=8*(u-k3)
  Gain1 : Gain  Gain=k2
  Product1 : Product  Inputs=3
  Product2 : Product
  Product3 : Product
  Sqrt1 : Sqrt
  k : Constant  Value=k
  q1 : Outport
  wires:
  Product3/1 -> Add1/2
  kn1/1 -> Product1/1, Product1/2, Gain1/1
  Constant/1 -> Divide/1
  Fcn3/1 -> Divide/2
  perturbatie k/1 -> Add2/1
  h1/1 -> Product3/2
  k/1 -> Add2/2
  Fcn4/1 -> Product3/1
  Divide/1 -> Product2/2
  Add/1 -> Product2/1
  Product1/1 -> Add1/1
  Product2/1 -> q1/1
  Add1/1 -> Sqrt1/1
  Add2/1 -> Fcn4/1, Fcn3/1, Fcn/1
  Gain1/1 -> Add/1
  Sqrt1/1 -> Add/2
  Fcn/1 -> Product1/3

== system ProiectSCPC_Reglare_Nivel/Subsystem4/Randament ==
  q : Inport
  um : Inport  Port=2
  Gain8 : Gain  Gain=keta
  Product1 : Product
  eta : Outport
  wires:
  um/1 -> Gain8/1
  Gain8/1 -> Product1/2
  q/1 -> Product1/1
  Product1/1 -> eta/1

== system ProiectSCPC_Reglare_Nivel/Subsystem4/Subsystem ==
  q : Inport
  Integrator : Integrator  InitialCondition=29.2
  Sum : Sum  Inputs=|+-
  h : Outport
  wires:
  q/1 -> Sum/1
  Integrator/1 -> h/1, Sum/2
  Sum/1 -> Integrator/1

== system ProiectSCPC_Reglare_Nivel/cascada/Amplificator  ==
  ua : Inport
  Constant : Constant  Value=8.1
  Gain : Gain  Gain=2.2
  Gain1 : Gain  Gain=5
  Gain2 : Gain  Gain=2.2
  Saturation : Saturate  UpperLimit=22  LowerLimit=0
  Sum : Sum  Inputs=|+-
  Sum1 : Sum  Inputs=|++
  Switch : Switch  Threshold=8.1  SaturateOnIntegerOverflow=off  InputSameDT=off
  um : Outport
  wires:
  Gain/1 -> Switch/3
  Gain1/1 -> Sum1/2
  Switch/1 -> Saturation/1
  Constant/1 -> Sum/2
  Gain2/1 -> Sum1/1
  Sum/1 -> Gain1/1
  Saturation/1 -> um/1
  ua/1 -> Sum/1, Gain2/1, Gain/1, Switch/2
  Sum1/1 -> Switch/1

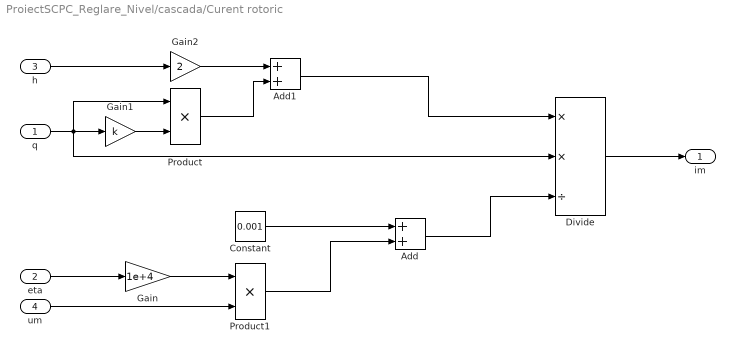
== system ProiectSCPC_Reglare_Nivel/cascada/Curent rotoric ==
  q : Inport
  eta : Inport  Port=2
  h : Inport  Port=3
  um : Inport  Port=4
  Add : Sum
  Add1 : Sum
  Constant : Constant  Value=0.001
  Divide : Product  Inputs=**/
  Gain : Gain  Gain=1e+4
  Gain1 : Gain  Gain=k
  Gain2 : Gain  Gain=2
  Product : Product
  Product1 : Product
  im : Outport
  wires:
  Add1/1 -> Divide/1
  Constant/1 -> Add/1
  Add/1 -> Divide/3
  Gain1/1 -> Product/2
  Product/1 -> Add1/2
  um/1 -> Product1/2
  Product1/1 -> Add/2
  Divide/1 -> im/1
  Gain/1 -> Product1/1
  Gain2/1 -> Add1/1
  eta/1 -> Gain/1
  q/1 -> Divide/2, Product/1, Gain1/1
  h/1 -> Gain2/1

== system ProiectSCPC_Reglare_Nivel/cascada/Filtru ==
  q : Inport
  Integrator : Integrator  InitialCondition=29.2
  Sum : Sum  Inputs=|+-
  h : Outport
  wires:
  Sum/1 -> Integrator/1
  q/1 -> Sum/1
  Integrator/1 -> h/1, Sum/2

== system ProiectSCPC_Reglare_Nivel/cascada/Motor ==
  um : Inport
  im : Inport  Port=2
  Add : Sum  Inputs=+-
  "Rm " : Gain  Gain=3
  kn : Outport
  wires:
  "Rm "/1 -> Add/2
  Add/1 -> kn/1
  um/1 -> Add/1
  im/1 -> "Rm "/1

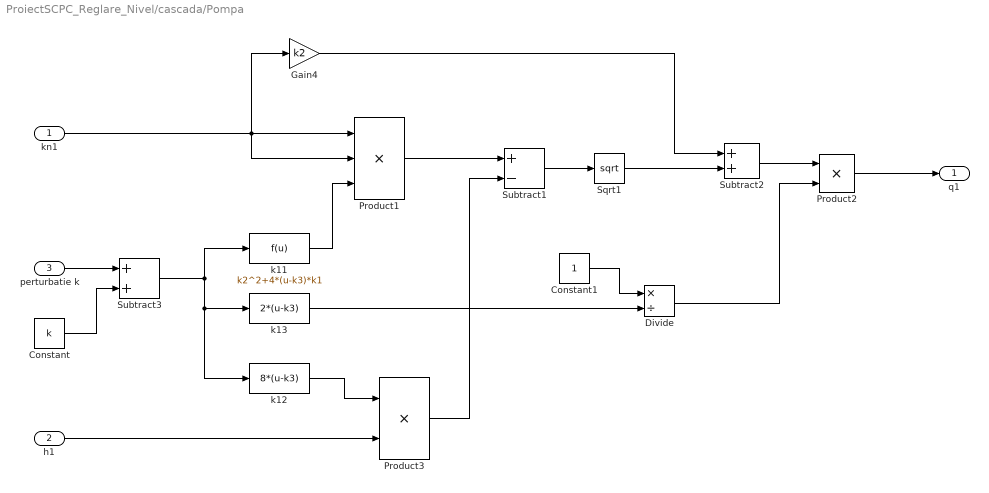
== system ProiectSCPC_Reglare_Nivel/cascada/Pompa ==
  kn1 : Inport
  h1 : Inport  Port=2
  perturbatie k : Inport  Port=3
  Constant : Constant  Value=k
  Constant1 : Constant
  Divide : Product  Inputs=*/
  Gain4 : Gain  Gain=k2
  Product1 : Product  Inputs=3
  Product2 : Product
  Product3 : Product
  Sqrt1 : Sqrt
  Subtract1 : Sum  Inputs=+-
  Subtract2 : Sum
  Subtract3 : Sum
  k11 : Fcn  Expr=k2^2+4*(u-k3)*k1
  k12 : Fcn  Expr=8*(u-k3)
  k13 : Fcn  Expr=2*(u-k3)
  q1 : Outport
  wires:
  kn1/1 -> Gain4/1, Product1/1, Product1/2
  Subtract1/1 -> Sqrt1/1
  Gain4/1 -> Subtract2/1
  Sqrt1/1 -> Subtract2/2
  perturbatie k/1 -> Subtract3/1
  Constant/1 -> Subtract3/2
  Product2/1 -> q1/1
  Subtract2/1 -> Product2/1
  Divide/1 -> Product2/2
  Constant1/1 -> Divide/1
  Product1/1 -> Subtract1/1
  h1/1 -> Product3/2
  Product3/1 -> Subtract1/2
  k11/1 -> Product1/3
  Subtract3/1 -> k12/1, k13/1, k11/1
  k12/1 -> Product3/1
  k13/1 -> Divide/2

== system ProiectSCPC_Reglare_Nivel/cascada/Randament ==
  q : Inport
  um : Inport  Port=2
  Gain : Gain  Gain=keta
  Product : Product
  eta : Outport
  wires:
  Gain/1 -> Product/2
  Product/1 -> eta/1
  q/1 -> Product/1
  um/1 -> Gain/1

== system ProiectSCPC_Reglare_Nivel/cascada/Rezervor ==
  q : Inport
  Fcn : Fcn  Expr=sqrt(u)*9
  Gain : Gain  Gain=1/332.5
  Integrator : Integrator  InitialCondition=10.5
  Sum : Sum  Inputs=|+-
  h : Outport
  wires:
  q/1 -> Sum/1
  Sum/1 -> Gain/1
  Integrator/1 -> h/1, Fcn/1
  Fcn/1 -> Sum/2
  Gain/1 -> Integrator/1

== system ProiectSCPC_Reglare_Nivel/cascada si feed-forward/Amplificator  ==
  ua : Inport
  Constant : Constant  Value=8.1
  Gain : Gain  Gain=2.2
  Gain1 : Gain  Gain=5
  Gain2 : Gain  Gain=2.2
  Saturation : Saturate  UpperLimit=22  LowerLimit=0
  Sum : Sum  Inputs=|+-
  Sum1 : Sum  Inputs=|++
  Switch : Switch  Threshold=8.1  SaturateOnIntegerOverflow=off  InputSameDT=off
  um : Outport
  wires:
  Gain/1 -> Switch/3
  Gain1/1 -> Sum1/2
  Switch/1 -> Saturation/1
  Constant/1 -> Sum/2
  Gain2/1 -> Sum1/1
  Sum/1 -> Gain1/1
  Saturation/1 -> um/1
  ua/1 -> Sum/1, Gain2/1, Gain/1, Switch/2
  Sum1/1 -> Switch/1

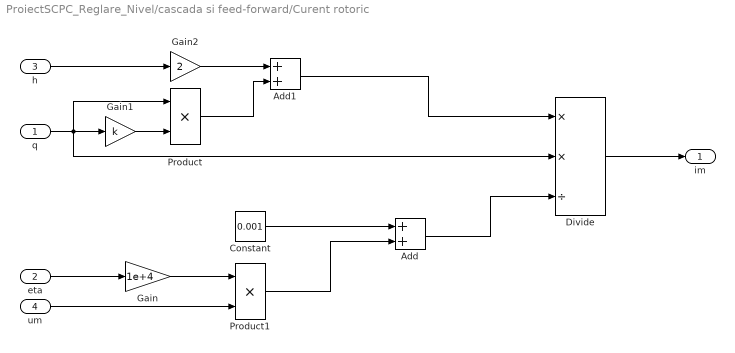
== system ProiectSCPC_Reglare_Nivel/cascada si feed-forward/Curent rotoric ==
  q : Inport
  eta : Inport  Port=2
  h : Inport  Port=3
  um : Inport  Port=4
  Add : Sum
  Add1 : Sum
  Constant : Constant  Value=0.001
  Divide : Product  Inputs=**/
  Gain : Gain  Gain=1e+4
  Gain1 : Gain  Gain=k
  Gain2 : Gain  Gain=2
  Product : Product
  Product1 : Product
  im : Outport
  wires:
  Add1/1 -> Divide/1
  Constant/1 -> Add/1
  Add/1 -> Divide/3
  Gain1/1 -> Product/2
  Product/1 -> Add1/2
  um/1 -> Product1/2
  Product1/1 -> Add/2
  Divide/1 -> im/1
  Gain/1 -> Product1/1
  Gain2/1 -> Add1/1
  eta/1 -> Gain/1
  q/1 -> Divide/2, Product/1, Gain1/1
  h/1 -> Gain2/1

== system ProiectSCPC_Reglare_Nivel/cascada si feed-forward/Filtru ==
  q : Inport
  Integrator : Integrator  InitialCondition=29.2
  Sum : Sum  Inputs=|+-
  h : Outport
  wires:
  Sum/1 -> Integrator/1
  q/1 -> Sum/1
  Integrator/1 -> h/1, Sum/2

== system ProiectSCPC_Reglare_Nivel/cascada si feed-forward/Motor ==
  um : Inport
  im : Inport  Port=2
  Add : Sum  Inputs=+-
  "Rm " : Gain  Gain=3
  kn : Outport
  wires:
  "Rm "/1 -> Add/2
  Add/1 -> kn/1
  um/1 -> Add/1
  im/1 -> "Rm "/1

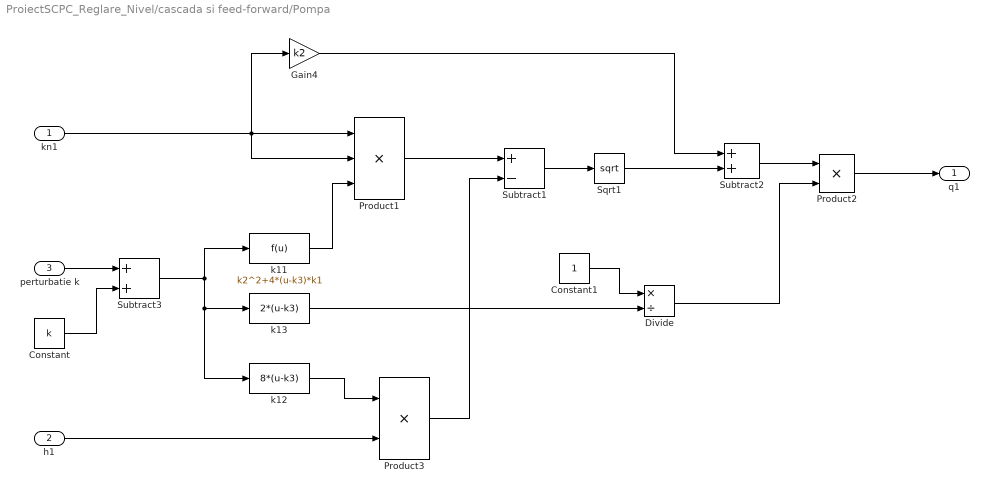
== system ProiectSCPC_Reglare_Nivel/cascada si feed-forward/Pompa ==
  kn1 : Inport
  h1 : Inport  Port=2
  perturbatie k : Inport  Port=3
  Constant : Constant  Value=k
  Constant1 : Constant
  Divide : Product  Inputs=*/
  Gain4 : Gain  Gain=k2
  Product1 : Product  Inputs=3
  Product2 : Product
  Product3 : Product
  Sqrt1 : Sqrt
  Subtract1 : Sum  Inputs=+-
  Subtract2 : Sum
  Subtract3 : Sum
  k11 : Fcn  Expr=k2^2+4*(u-k3)*k1
  k12 : Fcn  Expr=8*(u-k3)
  k13 : Fcn  Expr=2*(u-k3)
  q1 : Outport
  wires:
  kn1/1 -> Gain4/1, Product1/1, Product1/2
  Subtract1/1 -> Sqrt1/1
  Gain4/1 -> Subtract2/1
  Sqrt1/1 -> Subtract2/2
  perturbatie k/1 -> Subtract3/1
  Constant/1 -> Subtract3/2
  Product2/1 -> q1/1
  Subtract2/1 -> Product2/1
  Divide/1 -> Product2/2
  Constant1/1 -> Divide/1
  Product1/1 -> Subtract1/1
  h1/1 -> Product3/2
  Product3/1 -> Subtract1/2
  k11/1 -> Product1/3
  Subtract3/1 -> k12/1, k13/1, k11/1
  k12/1 -> Product3/1
  k13/1 -> Divide/2

== system ProiectSCPC_Reglare_Nivel/cascada si feed-forward/Randament ==
  q : Inport
  um : Inport  Port=2
  Gain : Gain  Gain=keta
  Product : Product
  eta : Outport
  wires:
  Gain/1 -> Product/2
  Product/1 -> eta/1
  q/1 -> Product/1
  um/1 -> Gain/1

== system ProiectSCPC_Reglare_Nivel/cascada si feed-forward/Rezervor ==
  q : Inport
  Fcn : Fcn  Expr=sqrt(u)*9
  Gain : Gain  Gain=1/332.5
  Integrator : Integrator  InitialCondition=10.5
  Sum : Sum  Inputs=|+-
  h : Outport
  wires:
  q/1 -> Sum/1
  Sum/1 -> Gain/1
  Integrator/1 -> h/1, Fcn/1
  Fcn/1 -> Sum/2
  Gain/1 -> Integrator/1
